simulink model "xtao"  (Simulink 7.0)
settings: Solver=FixedStepDiscrete  SolverMode=SingleTasking  StartTime=0.0  StopTime=inf  FixedStep=0.002  RelTol=1e-3
undefined symbols (not defined in the file): fdesignblkfcn, gcbh, HIL
libraries: dspsigops x27, quarc_library x6
settings Model: Creator=Administrator  LastModifiedBy=Administrator  SimulationMode=external  ExtModeTrigDuration=5000
settings SolverCC: PositivePriorityOrder=on
settings DataIOCC: ExternalInput=[a1, a2]
settings RTWCC: SystemTargetFile=quarc_windows.tlc  TemplateMakefile=quarc_default_tmf  Description=QUARC Win32 Target  ProcessScript=quarc_windows_make_rtw_hook
settings STFCustomTargetCC: TargetPreCompLibLocation=C:\DOCUME~1\ALLUSE~1\APPLIC~1\QUARC\lib\2007b\windows\release  GenFloatMathFcnCalls=ANSI_C  SystemTargetFile=quarc_windows.tlc
settings GRTTargetCC: TargetPreCompLibLocation=C:\DOCUME~1\ALLUSE~1\APPLIC~1\QUARC\lib\2007b\windows\release  CompOptLevelCompliant=off  MatFileLogging=off  ExtMode=on  ExtModeMexFile=quarc_comm

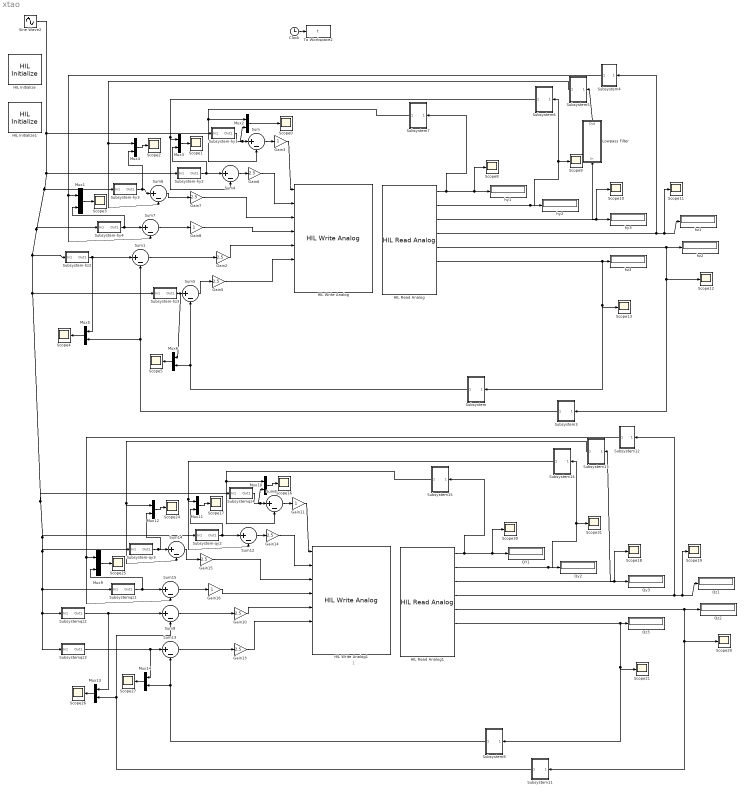
== system xtao ==
  note: 1
  Clock : Clock
      settings: Decimation=10
  Gain{2,5..7,10,13..15} (8 alike) : Gain  Gain=2.5  ParameterDataType=sfix(16)  ParameterScaling=2^0  OutDataType=sfix(16)  OutScaling=2^0
  Gain{3,8,11,16} (4 alike) : Gain  ParameterDataType=sfix(16)  ParameterScaling=2^0  OutDataType=sfix(16)  OutScaling=2^0
  HIL Initialize : quarc_library/Data Acquisition/Generic/Configuration/HIL Initialize  object_name=HIL-1  board_type=qpid  board_number=0  board_options=enc0_dir=0;enc0_filter=1;enc0_a=1;enc0_b=1;enc0_z=0;enc0_reload=0;enc1_dir=0;enc1_filter=1;enc1_a=1;enc1_b=1;enc1_z=0;enc1_reload=0;enc2_dir=0;enc2_filter=1;enc2_a=1;enc2_b=1;enc2_z=0;enc2_reload=0;enc3_dir=0;enc3_filter=1;enc3_a=1;enc3_b=1;enc3_z=0;enc3_reload=0;enc4_dir=0;enc4_filter=1;enc4_a=1;enc4_b=1;enc4_z=0;enc4_reload=0;enc5_dir=0;enc5_filter=1;enc5_a=1;enc5_b=1;enc5_z=0;enc5_reload=0;enc6_dir=0;enc6_filter=1;enc6_a=1;enc6_b=1;enc6_z=0;enc6_reload=0;enc7_dir=0;enc7_filter=1;enc7_a=1;enc7_b=1;enc7_z=0;enc7_reload=0;ext_int_polarity=0;fuse_polarity=0;convert_polarity=0;watchdog_polarity=0;ext_int_watchdog=0;fuse_watchdog=0;trig1_watchdog=0;watchdog_to_trig1=0;watchdog_to_trig2=0;counter_to_trig0=0;trigger_adcs=0;latch_on_adc=0;pwm_immediate=0  exclusive=off  active=off  hardware_clocks=[0:16]  clock_modes=[]  set_clock_params_at_start=off  set_clock_params_at_switch_in=off  analog_input_channels=[0:7]  analog_input_maximums=10  analog_input_minimums=-10  set_analog_input_params_at_start=off  set_analog_input_params_at_switch_in=off  analog_output_channels=[0:7]  analog_output_maximums=10  analog_output_minimums=-10  initial_analog_outputs=[0]  final_analog_outputs=[0]  watchdog_analog_outputs=0  set_analog_output_params_at_start=off  set_analog_output_params_at_switch_in=off  set_analog_outputs_at_start=on  set_analog_outputs_at_switch_in=off  set_analog_outputs_at_terminate=on  set_analog_outputs_at_switch_out=off  set_analog_outputs_on_watchdog=off  digital_input_channels=[]  digital_output_channels=[]  digital_output_configuration=[]  initial_digital_outputs=[1]  final_digital_outputs=[1]  watchdog_digital_outputs=[2]  set_digital_output_params_at_start=off  set_digital_output_params_at_switch_in=off  set_digital_outputs_at_start=on  set_digital_outputs_at_switch_in=off  set_digital_outputs_at_terminate=on  set_digital_outputs_at_switch_out=off  set_digital_outputs_on_watchdog=off  encoder_channels=[0:7]  quadrature=[4]  encoder_filter_frequency=40e6/1  initial_encoder_counts=[0]  set_encoder_params_at_start=on  set_encoder_params_at_switch_in=off  set_encoder_counts_at_start=on  set_encoder_counts_at_switch_in=off  pwm_channels=[0:7]  pwm_modes=0  pwm_frequency=40e6/4095  pwm_configuration=[0]  pwm_alignment=[0]  pwm_polarity=[1]  pwm_leading_deadband=[0]  pwm_trailing_deadband=[0]  initial_pwm_outputs=[0]  final_pwm_outputs=[0]  watchdog_pwm_outputs=[0]  set_pwm_params_at_start=on  set_pwm_params_at_switch_in=off  set_pwm_outputs_at_start=on  set_pwm_outputs_at_switch_in=off  set_pwm_outputs_at_terminate=on  set_pwm_outputs_at_switch_out=off  set_pwm_outputs_on_watchdog=off  other_output_channels=[]  initial_other_outputs=[]  final_other_outputs=[]  watchdog_other_outputs=[]  set_other_outputs_at_start=off  set_other_outputs_at_switch_in=off  set_other_outputs_at_terminate=off  set_other_outputs_at_switch_out=off  set_other_outputs_on_watchdog=off
  HIL Initialize1 : quarc_library/Data Acquisition/Generic/Configuration/HIL Initialize  object_name=HIL-2  board_type=qpid  board_number=1  board_options=enc0_dir=0;enc0_filter=1;enc0_a=1;enc0_b=1;enc0_z=0;enc0_reload=0;enc1_dir=0;enc1_filter=1;enc1_a=1;enc1_b=1;enc1_z=0;enc1_reload=0;enc2_dir=0;enc2_filter=1;enc2_a=1;enc2_b=1;enc2_z=0;enc2_reload=0;enc3_dir=0;enc3_filter=1;enc3_a=1;enc3_b=1;enc3_z=0;enc3_reload=0;enc4_dir=0;enc4_filter=1;enc4_a=1;enc4_b=1;enc4_z=0;enc4_reload=0;enc5_dir=0;enc5_filter=1;enc5_a=1;enc5_b=1;enc5_z=0;enc5_reload=0;enc6_dir=0;enc6_filter=1;enc6_a=1;enc6_b=1;enc6_z=0;enc6_reload=0;enc7_dir=0;enc7_filter=1;enc7_a=1;enc7_b=1;enc7_z=0;enc7_reload=0;ext_int_polarity=0;fuse_polarity=0;convert_polarity=0;watchdog_polarity=0;ext_int_watchdog=0;fuse_watchdog=0;trig1_watchdog=0;watchdog_to_trig1=0;watchdog_to_trig2=0;counter_to_trig0=0;trigger_adcs=0;latch_on_adc=0;pwm_immediate=0  exclusive=off  active=off  hardware_clocks=[0:16]  clock_modes=[]  set_clock_params_at_start=off  set_clock_params_at_switch_in=off  analog_input_channels=[0:7]  analog_input_maximums=10  analog_input_minimums=-10  set_analog_input_params_at_start=off  set_analog_input_params_at_switch_in=off  analog_output_channels=[0:7]  analog_output_maximums=10  analog_output_minimums=-10  initial_analog_outputs=[0]  final_analog_outputs=[0]  watchdog_analog_outputs=0  set_analog_output_params_at_start=off  set_analog_output_params_at_switch_in=off  set_analog_outputs_at_start=on  set_analog_outputs_at_switch_in=off  set_analog_outputs_at_terminate=on  set_analog_outputs_at_switch_out=off  set_analog_outputs_on_watchdog=off  digital_input_channels=[]  digital_output_channels=[]  digital_output_configuration=[]  initial_digital_outputs=[1]  final_digital_outputs=[1]  watchdog_digital_outputs=[2]  set_digital_output_params_at_start=off  set_digital_output_params_at_switch_in=off  set_digital_outputs_at_start=on  set_digital_outputs_at_switch_in=off  set_digital_outputs_at_terminate=on  set_digital_outputs_at_switch_out=off  set_digital_outputs_on_watchdog=off  encoder_channels=[0:7]  quadrature=[4]  encoder_filter_frequency=40e6/1  initial_encoder_counts=[0]  set_encoder_params_at_start=on  set_encoder_params_at_switch_in=off  set_encoder_counts_at_start=on  set_encoder_counts_at_switch_in=off  pwm_channels=[0:7]  pwm_modes=0  pwm_frequency=40e6/4095  pwm_configuration=[0]  pwm_alignment=[0]  pwm_polarity=[1]  pwm_leading_deadband=[0]  pwm_trailing_deadband=[0]  initial_pwm_outputs=[0]  final_pwm_outputs=[0]  watchdog_pwm_outputs=[0]  set_pwm_params_at_start=on  set_pwm_params_at_switch_in=off  set_pwm_outputs_at_start=on  set_pwm_outputs_at_switch_in=off  set_pwm_outputs_at_terminate=on  set_pwm_outputs_at_switch_out=off  set_pwm_outputs_on_watchdog=off  other_output_channels=[]  initial_other_outputs=[]  final_other_outputs=[]  watchdog_other_outputs=[]  set_other_outputs_at_start=off  set_other_outputs_at_switch_in=off  set_other_outputs_at_terminate=off  set_other_outputs_at_switch_out=off  set_other_outputs_on_watchdog=off
  HIL Read Analog : quarc_library/Data Acquisition/Generic/Immediate I//O/HIL Read Analog  object_name=HIL-2  channels=[0:7]  sample_time=qc_get_step_size  active=on  vector_output=off
  HIL Read Analog1 : quarc_library/Data Acquisition/Generic/Immediate I//O/HIL Read Analog  object_name=HIL-1  channels=[0:7]  sample_time=qc_get_step_size  active=on  vector_output=off
  HIL Write Analog : quarc_library/Data Acquisition/Generic/Immediate I//O/HIL Write Analog  object_name=HIL-2  channels=[0:7]  sample_time=-1  active=off  vector_input=off
  HIL Write Analog1 : quarc_library/Data Acquisition/Generic/Immediate I//O/HIL Write Analog  object_name=HIL-1  channels=[0:7]  sample_time=-1  active=off  vector_input=off
  Lowpass Filter : Subsystem  Orientation=up  DialogController=fdesignblkfcn  DialogControllerArgs=DataTag7  InitFcn=fdesignblkfcn(gcbh, {'InitFcn'});
      settings: CopyFcn=fdesignblkfcn(gcbh, {'CopyFcn'});
      mask Type: Lowpass Filter
      mask Description: Design a lowpass filter
      mask Help: helpview(mapfilelocation('dspblks'), 'dsplowpassfilter')
      mask Display: disp('Lowpass')
  Mux{1..4,9..12} (8 alike) : Mux  Inputs=2
  Mux{5..6,13..14} (4 alike) : Mux  Orientation=left  Inputs=2
  QY1 : Display
  Qy2 : Display
  Qy3 : Display
  Qz1 : Display
  Qz2 : Display
  Qz3 : Display
  Scope{0..5,8..13,16..21,24..27,30..31} (24 alike) : Scope
      Scope0 settings: TimeRange=15  YMin=2  YMax=5.75  SaveName=ScopeData3  SampleInput=on
      Scope1 settings: TimeRange=15  YMin=0.5  YMax=4  SaveName=ScopeData4  SampleInput=on
      Scope10 settings: YMin=0.6  YMax=1.45  SaveName=ScopeData11
      Scope11 settings: YMin=1.045  YMax=1.065  SaveName=ScopeData2
      Scope12 settings: YMin=0.68175  YMax=0.68375  SaveName=ScopeData12
      Scope13 settings: YMin=0  YMax=2  SaveName=ScopeData13
      Scope16 settings: TimeRange=15  YMin=0.5  YMax=4.5  SaveName=ScopeData16  SampleInput=on
      Scope17 settings: TimeRange=15  YMin=0.5  YMax=4  SaveName=ScopeData17  SampleInput=on
      Scope18 settings: YMin=0.5  YMax=0.85  SaveName=ScopeData18
      Scope19 settings: YMin=0.7  YMax=1.3  SaveName=ScopeData19
      Scope2 settings: TimeRange=15  YMin=-0.5  YMax=5.25  SaveName=ScopeData5  SampleInput=on
      Scope20 settings: YMin=0.4  YMax=1.3  SaveName=ScopeData20
      Scope21 settings: YMin=0  YMax=2  SaveName=ScopeData21
      Scope24 settings: TimeRange=15  YMin=0.2  YMax=2.4  SaveName=ScopeData24  SampleInput=on
      Scope25 settings: TimeRange=15  YMin=0.3  YMax=2.1  SaveName=ScopeData25  SampleInput=on
      Scope26 settings: TimeRange=15  YMax=10  SaveName=ScopeData26  SampleInput=on
      Scope27 settings: TimeRange=15  YMin=1.975  YMax=2.4  SaveName=ScopeData27  SampleInput=on
      Scope3 settings: TimeRange=15  YMin=1.85  YMax=2.3  SampleInput=on
      Scope30 settings: YMin=-0.005  YMax=0.015  SaveName=ScopeData30
      Scope31 settings: YMin=-0.000305176  YMax=-0.000305176  SaveName=ScopeData31
      Scope4 settings: TimeRange=15  YMin=0.5  YMax=4  SaveName=ScopeData6  SampleInput=on
      Scope5 settings: TimeRange=15  YMin=-2.75  YMax=3  SaveName=ScopeData7  SampleInput=on
      Scope8 settings: TimeRange=10  YMin=0.8785  YMax=0.8875  SaveName=ScopeData9
      Scope9 settings: YMin=0.129  YMax=0.1307  SaveName=ScopeData10
  Sine Wave2 : Sin  Bias=20  Frequency=3.14  SampleTime=0
  Subsystem : Subsystem  Orientation=left
  Subsystem-hy1 : Subsystem
  Subsystem-hy2 : Subsystem
  Subsystem-hy3 : Subsystem
  Subsystem-hy4 : Subsystem
  Subsystem-hz2 : Subsystem
  Subsystem-hz3 : Subsystem
  Subsystem-qy2 : Subsystem
  Subsystem-qy3 : Subsystem
  Subsystem11 : Subsystem  Orientation=left
  Subsystem12 : Subsystem  Orientation=left
  Subsystem13 : Subsystem  Orientation=left
  Subsystem14 : Subsystem  Orientation=left
  Subsystem15 : Subsystem  Orientation=left
  Subsystem3 : Subsystem  Orientation=left
  Subsystem4 : Subsystem  Orientation=left
  Subsystem5 : Subsystem  Orientation=left
  Subsystem6 : Subsystem  Orientation=left
  Subsystem7 : Subsystem  Orientation=left
  Subsystem8 : Subsystem  Orientation=left
  Subsystemqz1 : Subsystem
  Subsystemqz2 : Subsystem
  Subsystemqz3 : Subsystem
  Subsystemqz4 : Subsystem
  Sum{,1,4..9,12..15} (12 alike) : Sum  Inputs=|+-  OutDataType=sfix(16)  OutScaling=2^0
  To Workspace2 : ToWorkspace  VariableName=t  SampleTime=-1  SaveFormat=Array
  hy1 : Display
  hy2 : Display
  hy3 : Display
  hz1 : Display
  hz2 : Display
  hz3 : Display
  wires:
  HIL Read Analog/1 -> Subsystem7/1(In1), hy1/1, Scope8/1
  HIL Read Analog/2 -> hy2/1, Subsystem6/1(In1), Scope9/1
  HIL Read Analog/3 -> hy3/1, Scope10/1, Lowpass Filter/1(In)
  HIL Read Analog/4 -> Subsystem4/1(In1), hz1/1, Scope11/1
  HIL Read Analog/5 -> hz2/1, Scope12/1, Subsystem3/1(In1)
  HIL Read Analog/6 -> hz3/1, Subsystem/1(In1), Scope13/1
  Gain8/1 -> HIL Write Analog/4
  Clock/1 -> To Workspace2/1
  Gain2/1 -> HIL Write Analog/5
  Gain5/1 -> HIL Write Analog/6
  Sum5/1 -> Gain5/1
  Subsystem/1(Out1) -> Sum5/2, Mux6/2
  Sum1/1 -> Gain2/1
  Subsystem3/1(Out1) -> Sum1/2, Mux5/2
  Sum/1 -> Gain3/1
  Subsystem-hy1/1(Out1) -> Sum/1, Mux2/2
  Sum4/1 -> Gain6/1
  Subsystem-hy2/1(Out1) -> Sum4/1, Mux3/2
  Sum6/1 -> Gain7/1
  Subsystem7/1(Out1) -> Sum/2, Mux2/1
  Subsystem6/1(Out1) -> Sum4/2, Mux3/1
  Subsystem5/1(Out1) -> Sum6/2, Mux4/1
  Subsystem4/1(Out1) -> Sum7/2, Mux1/1
  Sum7/1 -> Gain8/1
  Subsystem-hy4/1(Out1) -> Sum7/1, Mux1/2
  Mux1/1 -> Scope3/1
  Subsystem-hz2/1(Out1) -> Sum1/1, Mux5/1
  Subsystem-hz3/1(Out1) -> Sum5/1, Mux6/1
  Mux2/1 -> Scope0/1
  Gain3/1 -> HIL Write Analog/1
  Mux3/1 -> Scope1/1
  Mux4/1 -> Scope2/1
  Mux5/1 -> Scope4/1
  Mux6/1 -> Scope5/1
  HIL Read Analog1/1 -> Subsystem15/1(In1), QY1/1, Scope30/1
  HIL Read Analog1/2 -> Qy2/1, Subsystem14/1(In1), Scope31/1
  HIL Read Analog1/3 -> Qy3/1, Subsystem13/1(In1), Scope18/1
  HIL Read Analog1/4 -> Subsystem12/1(In1), Qz1/1, Scope19/1
  HIL Read Analog1/5 -> Qz2/1, Scope20/1, Subsystem11/1(In1)
  HIL Read Analog1/6 -> Qz3/1, Subsystem8/1(In1), Scope21/1
  Gain16/1 -> HIL Write Analog1/4
  Gain10/1 -> HIL Write Analog1/5
  Gain14/1 -> HIL Write Analog1/2
  Gain13/1 -> HIL Write Analog1/6
  Sum13/1 -> Gain13/1
  Subsystem8/1(Out1) -> Sum13/2, Mux14/2
  Sum9/1 -> Gain10/1
  Subsystem11/1(Out1) -> Sum9/2, Mux13/2
  Sum8/1 -> Gain11/1
  Subsystemqz4/1(Out1) -> Sum8/1, Mux10/2
  Sum12/1 -> Gain14/1
  Subsystem-qy2/1(Out1) -> Sum12/1, Mux11/2
  Sum14/1 -> Gain15/1
  Subsystem-qy3/1(Out1) -> Mux12/2, Sum14/1
  Subsystem15/1(Out1) -> Sum8/2, Mux10/1
  Subsystem14/1(Out1) -> Sum12/2, Mux11/1
  Subsystem13/1(Out1) -> Sum14/2, Mux12/1
  Subsystem12/1(Out1) -> Sum15/2, Mux9/1
  Sum15/1 -> Gain16/1
  Subsystemqz1/1(Out1) -> Sum15/1, Mux9/2
  Mux9/1 -> Scope25/1
  Subsystemqz2/1(Out1) -> Sum9/1, Mux13/1
  Subsystemqz3/1(Out1) -> Mux14/1, Sum13/1
  Mux10/1 -> Scope16/1
  Gain11/1 -> HIL Write Analog1/1
  Mux11/1 -> Scope17/1
  Mux12/1 -> Scope24/1
  Mux13/1 -> Scope26/1
  Mux14/1 -> Scope27/1
  Lowpass Filter/1(Out) -> Subsystem5/1(In1)
  Sine Wave2/1 -> Subsystem-hy2/1(In1), Subsystem-hy3/1(In1), Subsystem-hz2/1(In1), Subsystem-hz3/1(In1), Subsystem-qy2/1(In1), Subsystem-qy3/1(In1), Subsystemqz2/1(In1), Subsystemqz3/1(In1), Subsystemqz1/1(In1), Subsystemqz4/1(In1), Subsystem-hy4/1(In1), Subsystem-hy1/1(In1)
  Subsystem-hy3/1(Out1) -> Sum6/1, Mux4/2
  Gain15/1 -> HIL Write Analog1/3
  Gain6/1 -> HIL Write Analog/2
  Gain7/1 -> HIL Write Analog/3

== system xtao/Lowpass Filter ==
  In : Inport  OutDataType=sfix(16)  OutScaling=2^0
  Generated Filter Block : Subsystem  Tag=FilterWizardSubSystem
      settings: ErrorFcn=dspFilterRealizedInBasicElemsAlgLoopErrFcnCallback
  Out : Outport  OutDataType=sfix(16)  OutScaling=2^0
  wires:
  In/1 -> Generated Filter Block/1(Input)
  Generated Filter Block/1(Output) -> Out/1

== system xtao/Subsystem ==
  In1 : Inport  Orientation=left
  Constant9 : Constant  Orientation=left  Value=-3.9461  OutDataType=sfix(16)  OutScaling=2^0
  Gain4 : Gain  Orientation=left  Gain=6.2956  ParameterDataType=sfix(16)  ParameterScaling=2^0  OutDataType=sfix(16)  OutScaling=2^0
  Sum4 : Sum  Orientation=left  Inputs=|++  OutDataType=sfix(16)  OutScaling=2^0
  Out1 : Outport  Orientation=left
  wires:
  Constant9/1 -> Sum4/1
  Gain4/1 -> Sum4/2
  In1/1 -> Gain4/1
  Sum4/1 -> Out1/1

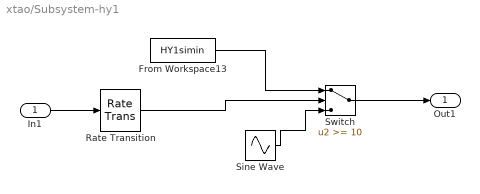
== system xtao/Subsystem-hy1 ==
  In1 : Inport  OutDataType=sfix(16)  OutScaling=2^0
  From Workspace13 : FromWorkspace  VariableName=HY1simin  SampleTime=0.01  Interpolate=off  OutputAfterFinalValue=Cyclic repetition
  Rate Transition : RateTransition
  Sine Wave : Sin  Amplitude=2.5  Bias=2.5  Frequency=3.14  SampleTime=0
  Switch : Switch  Threshold=10  OutDataType=sfix(16)  OutScaling=2^0
  Out1 : Outport  OutDataType=sfix(16)  OutScaling=2^0
  wires:
  From Workspace13/1 -> Switch/1
  Rate Transition/1 -> Switch/2
  Switch/1 -> Out1/1
  In1/1 -> Rate Transition/1
  Sine Wave/1 -> Switch/3

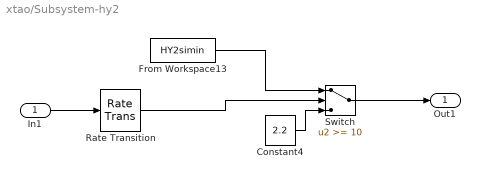
== system xtao/Subsystem-hy2 ==
  In1 : Inport  OutDataType=sfix(16)  OutScaling=2^0
  Constant4 : Constant  Value=2.2  OutDataType=sfix(16)  OutScaling=2^0
  From Workspace13 : FromWorkspace  VariableName=HY2simin  SampleTime=0.01  Interpolate=off  OutputAfterFinalValue=Cyclic repetition
  Rate Transition : RateTransition
  Switch : Switch  Threshold=10  OutDataType=sfix(16)  OutScaling=2^0
  Out1 : Outport  OutDataType=sfix(16)  OutScaling=2^0
  wires:
  From Workspace13/1 -> Switch/1
  Rate Transition/1 -> Switch/2
  Switch/1 -> Out1/1
  In1/1 -> Rate Transition/1
  Constant4/1 -> Switch/3

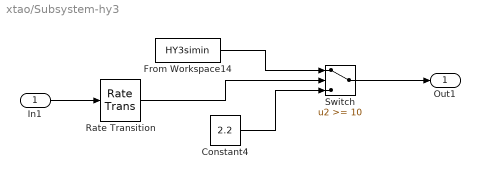
== system xtao/Subsystem-hy3 ==
  In1 : Inport  OutDataType=sfix(16)  OutScaling=2^0
  Constant4 : Constant  Value=2.2  OutDataType=sfix(16)  OutScaling=2^0
  From Workspace14 : FromWorkspace  VariableName=HY3simin  SampleTime=0.01  Interpolate=off  OutputAfterFinalValue=Cyclic repetition
  Rate Transition : RateTransition
  Switch : Switch  Threshold=10  OutDataType=sfix(16)  OutScaling=2^0
  Out1 : Outport  OutDataType=sfix(16)  OutScaling=2^0
  wires:
  Constant4/1 -> Switch/3
  From Workspace14/1 -> Switch/1
  Rate Transition/1 -> Switch/2
  Switch/1 -> Out1/1
  In1/1 -> Rate Transition/1

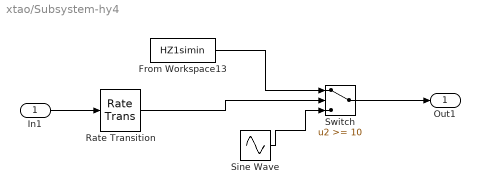
== system xtao/Subsystem-hy4 ==
  In1 : Inport  OutDataType=sfix(16)  OutScaling=2^0
  From Workspace13 : FromWorkspace  VariableName=HZ1simin  SampleTime=0.01  Interpolate=off  OutputAfterFinalValue=Cyclic repetition
  Rate Transition : RateTransition
  Sine Wave : Sin  Amplitude=2.5  Bias=2.5  Frequency=3.14  SampleTime=0
  Switch : Switch  Threshold=10  OutDataType=sfix(16)  OutScaling=2^0
  Out1 : Outport  OutDataType=sfix(16)  OutScaling=2^0
  wires:
  From Workspace13/1 -> Switch/1
  Rate Transition/1 -> Switch/2
  Switch/1 -> Out1/1
  In1/1 -> Rate Transition/1
  Sine Wave/1 -> Switch/3

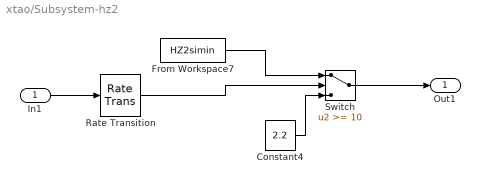
== system xtao/Subsystem-hz2 ==
  In1 : Inport  OutDataType=sfix(16)  OutScaling=2^0
  Constant4 : Constant  Value=2.2  OutDataType=sfix(16)  OutScaling=2^0
  From Workspace7 : FromWorkspace  VariableName=HZ2simin  SampleTime=0.01  Interpolate=off  OutputAfterFinalValue=Cyclic repetition
  Rate Transition : RateTransition
  Switch : Switch  Threshold=10  OutDataType=sfix(16)  OutScaling=2^0
  Out1 : Outport  OutDataType=sfix(16)  OutScaling=2^0
  wires:
  From Workspace7/1 -> Switch/1
  Rate Transition/1 -> Switch/2
  Switch/1 -> Out1/1
  In1/1 -> Rate Transition/1
  Constant4/1 -> Switch/3

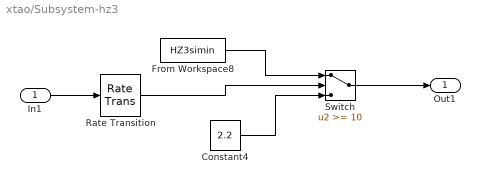
== system xtao/Subsystem-hz3 ==
  In1 : Inport  OutDataType=sfix(16)  OutScaling=2^0
  Constant4 : Constant  Value=2.2  OutDataType=sfix(16)  OutScaling=2^0
  From Workspace8 : FromWorkspace  VariableName=HZ3simin  SampleTime=0.01  Interpolate=off  OutputAfterFinalValue=Cyclic repetition
  Rate Transition : RateTransition
  Switch : Switch  Threshold=10  OutDataType=sfix(16)  OutScaling=2^0
  Out1 : Outport  OutDataType=sfix(16)  OutScaling=2^0
  wires:
  Constant4/1 -> Switch/3
  From Workspace8/1 -> Switch/1
  Rate Transition/1 -> Switch/2
  Switch/1 -> Out1/1
  In1/1 -> Rate Transition/1

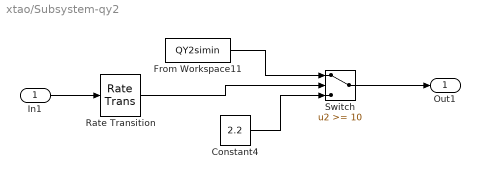
== system xtao/Subsystem-qy2 ==
  In1 : Inport  OutDataType=sfix(16)  OutScaling=2^0
  Constant4 : Constant  Value=2.2  OutDataType=sfix(16)  OutScaling=2^0
  From Workspace11 : FromWorkspace  VariableName=QY2simin  SampleTime=0.01  Interpolate=off  OutputAfterFinalValue=Cyclic repetition
  Rate Transition : RateTransition
  Switch : Switch  Threshold=10  OutDataType=sfix(16)  OutScaling=2^0
  Out1 : Outport  OutDataType=sfix(16)  OutScaling=2^0
  wires:
  Rate Transition/1 -> Switch/2
  Switch/1 -> Out1/1
  In1/1 -> Rate Transition/1
  From Workspace11/1 -> Switch/1
  Constant4/1 -> Switch/3

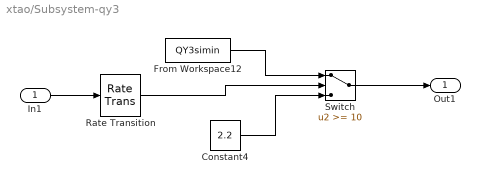
== system xtao/Subsystem-qy3 ==
  In1 : Inport  OutDataType=sfix(16)  OutScaling=2^0
  Constant4 : Constant  Value=2.2  OutDataType=sfix(16)  OutScaling=2^0
  From Workspace12 : FromWorkspace  VariableName=QY3simin  SampleTime=0.01  Interpolate=off  OutputAfterFinalValue=Cyclic repetition
  Rate Transition : RateTransition
  Switch : Switch  Threshold=10  OutDataType=sfix(16)  OutScaling=2^0
  Out1 : Outport  OutDataType=sfix(16)  OutScaling=2^0
  wires:
  Constant4/1 -> Switch/3
  From Workspace12/1 -> Switch/1
  Rate Transition/1 -> Switch/2
  Switch/1 -> Out1/1
  In1/1 -> Rate Transition/1

== system xtao/Subsystem11 ==
  In1 : Inport  Orientation=left
  Constant9 : Constant  Orientation=left  Value=-4.0345  OutDataType=sfix(16)  OutScaling=2^0
  Gain4 : Gain  Orientation=left  Gain=7.5666  ParameterDataType=sfix(16)  ParameterScaling=2^0  OutDataType=sfix(16)  OutScaling=2^0
  Sum4 : Sum  Orientation=left  Inputs=|++  OutDataType=sfix(16)  OutScaling=2^0
  Out1 : Outport  Orientation=left
  wires:
  Constant9/1 -> Sum4/1
  Gain4/1 -> Sum4/2
  In1/1 -> Gain4/1
  Sum4/1 -> Out1/1

== system xtao/Subsystem12 ==
  In1 : Inport  Orientation=left
  Constant9 : Constant  Orientation=left  Value=44.9691  OutDataType=sfix(16)  OutScaling=2^0
  Gain4 : Gain  Orientation=left  Gain=-10.3093  ParameterDataType=sfix(16)  ParameterScaling=2^0  OutDataType=sfix(16)  OutScaling=2^0
  Sum4 : Sum  Orientation=left  Inputs=|++  OutDataType=sfix(16)  OutScaling=2^0
  Out1 : Outport  Orientation=left
  wires:
  Constant9/1 -> Sum4/1
  Gain4/1 -> Sum4/2
  In1/1 -> Gain4/1
  Sum4/1 -> Out1/1

== system xtao/Subsystem13 ==
  In1 : Inport  Orientation=left
  Constant9 : Constant  Orientation=left  Value=-3.3411  OutDataType=sfix(16)  OutScaling=2^0
  Gain4 : Gain  Orientation=left  Gain=6.6836  ParameterDataType=sfix(16)  ParameterScaling=2^0  OutDataType=sfix(16)  OutScaling=2^0
  Sum4 : Sum  Orientation=left  Inputs=|++  OutDataType=sfix(16)  OutScaling=2^0
  Out1 : Outport  Orientation=left
  wires:
  Constant9/1 -> Sum4/1
  Gain4/1 -> Sum4/2
  In1/1 -> Gain4/1
  Sum4/1 -> Out1/1

== system xtao/Subsystem14 ==
  In1 : Inport  Orientation=left
  Constant9 : Constant  Orientation=left  Value=-3.8142  OutDataType=sfix(16)  OutScaling=2^0
  Gain4 : Gain  Orientation=left  Gain=7.9479  ParameterDataType=sfix(16)  ParameterScaling=2^0  OutDataType=sfix(16)  OutScaling=2^0
  Sum4 : Sum  Orientation=left  Inputs=|++  OutDataType=sfix(16)  OutScaling=2^0
  Out1 : Outport  Orientation=left
  wires:
  Constant9/1 -> Sum4/1
  Gain4/1 -> Sum4/2
  In1/1 -> Gain4/1
  Sum4/1 -> Out1/1

== system xtao/Subsystem15 ==
  In1 : Inport  Orientation=left
  Constant9 : Constant  Orientation=left  Value=-3.4379  OutDataType=sfix(16)  OutScaling=2^0
  Gain4 : Gain  Orientation=left  Gain=8.6655  ParameterDataType=sfix(16)  ParameterScaling=2^0  OutDataType=sfix(16)  OutScaling=2^0
  Sum4 : Sum  Orientation=left  Inputs=|++  OutDataType=sfix(16)  OutScaling=2^0
  Out1 : Outport  Orientation=left
  wires:
  Constant9/1 -> Sum4/1
  Gain4/1 -> Sum4/2
  In1/1 -> Gain4/1
  Sum4/1 -> Out1/1

== system xtao/Subsystem3 ==
  In1 : Inport  Orientation=left
  Constant9 : Constant  Orientation=left  Value=-3.8231  OutDataType=sfix(16)  OutScaling=2^0
  Gain4 : Gain  Orientation=left  Gain=6.6489  ParameterDataType=sfix(16)  ParameterScaling=2^0  OutDataType=sfix(16)  OutScaling=2^0
  Sum4 : Sum  Orientation=left  Inputs=|++  OutDataType=sfix(16)  OutScaling=2^0
  Out1 : Outport  Orientation=left
  wires:
  Constant9/1 -> Sum4/1
  Gain4/1 -> Sum4/2
  In1/1 -> Gain4/1
  Sum4/1 -> Out1/1

== system xtao/Subsystem4 ==
  In1 : Inport  Orientation=left
  Constant9 : Constant  Orientation=left  Value=46.9136  OutDataType=sfix(16)  OutScaling=2^0
  Gain4 : Gain  Orientation=left  Gain=-10.2881  ParameterDataType=sfix(16)  ParameterScaling=2^0  OutDataType=sfix(16)  OutScaling=2^0
  Sum4 : Sum  Orientation=left  Inputs=|++  OutDataType=sfix(16)  OutScaling=2^0
  Out1 : Outport  Orientation=left
  wires:
  Constant9/1 -> Sum4/1
  Gain4/1 -> Sum4/2
  In1/1 -> Gain4/1
  Sum4/1 -> Out1/1

== system xtao/Subsystem5 ==
  In1 : Inport  Orientation=left
  Constant9 : Constant  Orientation=left  Value=-3.7624  OutDataType=sfix(16)  OutScaling=2^0
  Gain4 : Gain  Orientation=left  Gain=6.2189  ParameterDataType=sfix(16)  ParameterScaling=2^0  OutDataType=sfix(16)  OutScaling=2^0
  Sum4 : Sum  Orientation=left  Inputs=|++  OutDataType=sfix(16)  OutScaling=2^0
  Out1 : Outport  Orientation=left
  wires:
  Constant9/1 -> Sum4/1
  Gain4/1 -> Sum4/2
  In1/1 -> Gain4/1
  Sum4/1 -> Out1/1

== system xtao/Subsystem6 ==
  In1 : Inport  Orientation=left
  Constant9 : Constant  Orientation=left  Value=-4.6642  OutDataType=sfix(16)  OutScaling=2^0
  Gain4 : Gain  Orientation=left  Gain=7.4627  ParameterDataType=sfix(16)  ParameterScaling=2^0  OutDataType=sfix(16)  OutScaling=2^0
  Sum4 : Sum  Orientation=left  Inputs=|++  OutDataType=sfix(16)  OutScaling=2^0
  Out1 : Outport  Orientation=left
  wires:
  Constant9/1 -> Sum4/1
  Gain4/1 -> Sum4/2
  In1/1 -> Gain4/1
  Sum4/1 -> Out1/1

== system xtao/Subsystem7 ==
  In1 : Inport  Orientation=left
  Constant9 : Constant  Orientation=left  Value=-5.1224  OutDataType=sfix(16)  OutScaling=2^0
  Gain4 : Gain  Orientation=left  Gain=8.7413  ParameterDataType=sfix(16)  ParameterScaling=2^0  OutDataType=sfix(16)  OutScaling=2^0
  Sum4 : Sum  Orientation=left  Inputs=|++  OutDataType=sfix(16)  OutScaling=2^0
  Out1 : Outport  Orientation=left
  wires:
  Constant9/1 -> Sum4/1
  Gain4/1 -> Sum4/2
  In1/1 -> Gain4/1
  Sum4/1 -> Out1/1

== system xtao/Subsystem8 ==
  In1 : Inport  Orientation=left
  Constant9 : Constant  Orientation=left  Value=-3.1294  OutDataType=sfix(16)  OutScaling=2^0
  Gain4 : Gain  Orientation=left  Gain=6.7240  ParameterDataType=sfix(16)  ParameterScaling=2^0  OutDataType=sfix(16)  OutScaling=2^0
  Sum4 : Sum  Orientation=left  Inputs=|++  OutDataType=sfix(16)  OutScaling=2^0
  Out1 : Outport  Orientation=left
  wires:
  Constant9/1 -> Sum4/1
  Gain4/1 -> Sum4/2
  In1/1 -> Gain4/1
  Sum4/1 -> Out1/1

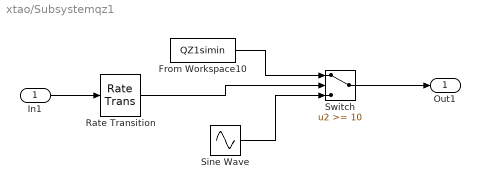
== system xtao/Subsystemqz1 ==
  In1 : Inport  OutDataType=sfix(16)  OutScaling=2^0
  From Workspace10 : FromWorkspace  VariableName=QZ1simin  SampleTime=0.01  Interpolate=off  OutputAfterFinalValue=Cyclic repetition
  Rate Transition : RateTransition
  Sine Wave : Sin  Amplitude=2.5  Bias=2.5  Frequency=3.14  SampleTime=0
  Switch : Switch  Threshold=10  OutDataType=sfix(16)  OutScaling=2^0
  Out1 : Outport  OutDataType=sfix(16)  OutScaling=2^0
  wires:
  Sine Wave/1 -> Switch/3
  From Workspace10/1 -> Switch/1
  Rate Transition/1 -> Switch/2
  Switch/1 -> Out1/1
  In1/1 -> Rate Transition/1

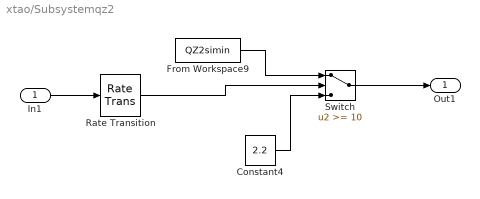
== system xtao/Subsystemqz2 ==
  In1 : Inport  OutDataType=sfix(16)  OutScaling=2^0
  Constant4 : Constant  Value=2.2  OutDataType=sfix(16)  OutScaling=2^0
  From Workspace9 : FromWorkspace  VariableName=QZ2simin  SampleTime=0.01  Interpolate=off  OutputAfterFinalValue=Cyclic repetition
  Rate Transition : RateTransition
  Switch : Switch  Threshold=10  OutDataType=sfix(16)  OutScaling=2^0
  Out1 : Outport  OutDataType=sfix(16)  OutScaling=2^0
  wires:
  From Workspace9/1 -> Switch/1
  Rate Transition/1 -> Switch/2
  Switch/1 -> Out1/1
  In1/1 -> Rate Transition/1
  Constant4/1 -> Switch/3

== system xtao/Subsystemqz3 ==
  In1 : Inport  OutDataType=sfix(16)  OutScaling=2^0
  Constant4 : Constant  Value=2.2  OutDataType=sfix(16)  OutScaling=2^0
  From Workspace10 : FromWorkspace  VariableName=QZ3simin  SampleTime=0.01  Interpolate=off  OutputAfterFinalValue=Cyclic repetition
  Rate Transition : RateTransition
  Switch : Switch  Threshold=10  OutDataType=sfix(16)  OutScaling=2^0
  Out1 : Outport  OutDataType=sfix(16)  OutScaling=2^0
  wires:
  Constant4/1 -> Switch/3
  From Workspace10/1 -> Switch/1
  Rate Transition/1 -> Switch/2
  Switch/1 -> Out1/1
  In1/1 -> Rate Transition/1

== system xtao/Subsystemqz4 ==
  In1 : Inport  OutDataType=sfix(16)  OutScaling=2^0
  From Workspace10 : FromWorkspace  VariableName=QY1simin  SampleTime=0.01  Interpolate=off  OutputAfterFinalValue=Cyclic repetition
  Rate Transition : RateTransition
  Sine Wave : Sin  Amplitude=2.5  Bias=2.5  Frequency=3.14  SampleTime=0
  Switch : Switch  Threshold=10  OutDataType=sfix(16)  OutScaling=2^0
  Out1 : Outport  OutDataType=sfix(16)  OutScaling=2^0
  wires:
  In1/1 -> Rate Transition/1
  Switch/1 -> Out1/1
  Rate Transition/1 -> Switch/2
  From Workspace10/1 -> Switch/1
  Sine Wave/1 -> Switch/3

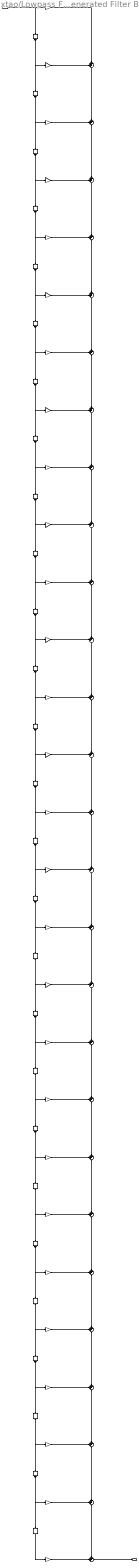
== system xtao/Lowpass Filter/Generated Filter Block ==
  Input : Inport
  BodyDelay{2..28} (27 alike) : dspsigops/Delay  Orientation=down  dly_unit=Samples  delay=1  ic_detail=off  dif_ic_for_ch=off  dif_ic_for_dly=off  ic=0  reset_popup=None
  BodyLSum{2..27} (26 alike) : Sum  Orientation=down  Inputs=++|  OutScaling=1  RndMeth=Nearest  SaturateOnIntegerOverflow=on
  BodyLSum28 : Sum  Inputs=++|  OutScaling=1  RndMeth=Nearest  SaturateOnIntegerOverflow=on
  b(1) : Gain  Gain=0.0030532375936556358  ParameterDataTypeMode=Specify via dialog  ParameterDataType=float('double')  ParameterScalingMode=Use specified scaling  ParameterScaling=1  OutScaling=1  RndMeth=Nearest  SaturateOnIntegerOverflow=on
  b(10) : Gain  Gain=-0.051710781607074402  ParameterDataTypeMode=Specify via dialog  ParameterDataType=float('double')  ParameterScalingMode=Use specified scaling  ParameterScaling=1  OutScaling=1  RndMeth=Nearest  SaturateOnIntegerOverflow=on
  b(11) : Gain  Gain=-0.071497034579946883  ParameterDataTypeMode=Specify via dialog  ParameterDataType=float('double')  ParameterScalingMode=Use specified scaling  ParameterScaling=1  OutScaling=1  RndMeth=Nearest  SaturateOnIntegerOverflow=on
  b(12) : Gain  Gain=0.021409500242294495  ParameterDataTypeMode=Specify via dialog  ParameterDataType=float('double')  ParameterScalingMode=Use specified scaling  ParameterScaling=1  OutScaling=1  RndMeth=Nearest  SaturateOnIntegerOverflow=on
  b(13) : Gain  Gain=0.20428929463408604  ParameterDataTypeMode=Specify via dialog  ParameterDataType=float('double')  ParameterScalingMode=Use specified scaling  ParameterScaling=1  OutScaling=1  RndMeth=Nearest  SaturateOnIntegerOverflow=on
  b(14) : Gain  Gain=0.3545770243381996  ParameterDataTypeMode=Specify via dialog  ParameterDataType=float('double')  ParameterScalingMode=Use specified scaling  ParameterScaling=1  OutScaling=1  RndMeth=Nearest  SaturateOnIntegerOverflow=on
  b(15) : Gain  Gain=0.3545770243381996  ParameterDataTypeMode=Specify via dialog  ParameterDataType=float('double')  ParameterScalingMode=Use specified scaling  ParameterScaling=1  OutScaling=1  RndMeth=Nearest  SaturateOnIntegerOverflow=on
  b(16) : Gain  Gain=0.20428929463408604  ParameterDataTypeMode=Specify via dialog  ParameterDataType=float('double')  ParameterScalingMode=Use specified scaling  ParameterScaling=1  OutScaling=1  RndMeth=Nearest  SaturateOnIntegerOverflow=on
  b(17) : Gain  Gain=0.021409500242294495  ParameterDataTypeMode=Specify via dialog  ParameterDataType=float('double')  ParameterScalingMode=Use specified scaling  ParameterScaling=1  OutScaling=1  RndMeth=Nearest  SaturateOnIntegerOverflow=on
  b(18) : Gain  Gain=-0.071497034579946883  ParameterDataTypeMode=Specify via dialog  ParameterDataType=float('double')  ParameterScalingMode=Use specified scaling  ParameterScaling=1  OutScaling=1  RndMeth=Nearest  SaturateOnIntegerOverflow=on
  b(19) : Gain  Gain=-0.051710781607074402  ParameterDataTypeMode=Specify via dialog  ParameterDataType=float('double')  ParameterScalingMode=Use specified scaling  ParameterScaling=1  OutScaling=1  RndMeth=Nearest  SaturateOnIntegerOverflow=on
  b(2) : Gain  Gain=0.0066380134927875832  ParameterDataTypeMode=Specify via dialog  ParameterDataType=float('double')  ParameterScalingMode=Use specified scaling  ParameterScaling=1  OutScaling=1  RndMeth=Nearest  SaturateOnIntegerOverflow=on
  b(20) : Gain  Gain=0.0090330088298889565  ParameterDataTypeMode=Specify via dialog  ParameterDataType=float('double')  ParameterScalingMode=Use specified scaling  ParameterScaling=1  OutScaling=1  RndMeth=Nearest  SaturateOnIntegerOverflow=on
  b(21) : Gain  Gain=0.034704857949413304  ParameterDataTypeMode=Specify via dialog  ParameterDataType=float('double')  ParameterScalingMode=Use specified scaling  ParameterScaling=1  OutScaling=1  RndMeth=Nearest  SaturateOnIntegerOverflow=on
  b(22) : Gain  Gain=0.013219031256279611  ParameterDataTypeMode=Specify via dialog  ParameterDataType=float('double')  ParameterScalingMode=Use specified scaling  ParameterScaling=1  OutScaling=1  RndMeth=Nearest  SaturateOnIntegerOverflow=on
  b(23) : Gain  Gain=-0.017112476184483319  ParameterDataTypeMode=Specify via dialog  ParameterDataType=float('double')  ParameterScalingMode=Use specified scaling  ParameterScaling=1  OutScaling=1  RndMeth=Nearest  SaturateOnIntegerOverflow=on
  b(24) : Gain  Gain=-0.024022228586093927  ParameterDataTypeMode=Specify via dialog  ParameterDataType=float('double')  ParameterScalingMode=Use specified scaling  ParameterScaling=1  OutScaling=1  RndMeth=Nearest  SaturateOnIntegerOverflow=on
  b(25) : Gain  Gain=-0.010230117696056244  ParameterDataTypeMode=Specify via dialog  ParameterDataType=float('double')  ParameterScalingMode=Use specified scaling  ParameterScaling=1  OutScaling=1  RndMeth=Nearest  SaturateOnIntegerOverflow=on
  b(26) : Gain  Gain=0.0036501248931968783  ParameterDataTypeMode=Specify via dialog  ParameterDataType=float('double')  ParameterScalingMode=Use specified scaling  ParameterScaling=1  OutScaling=1  RndMeth=Nearest  SaturateOnIntegerOverflow=on
  b(27) : Gain  Gain=0.0066380134927875832  ParameterDataTypeMode=Specify via dialog  ParameterDataType=float('double')  ParameterScalingMode=Use specified scaling  ParameterScaling=1  OutScaling=1  RndMeth=Nearest  SaturateOnIntegerOverflow=on
  b(28) : Gain  Gain=0.0030532375936556358  ParameterDataTypeMode=Specify via dialog  ParameterDataType=float('double')  ParameterScalingMode=Use specified scaling  ParameterScaling=1  OutScaling=1  RndMeth=Nearest  SaturateOnIntegerOverflow=on
  b(3) : Gain  Gain=0.0036501248931968783  ParameterDataTypeMode=Specify via dialog  ParameterDataType=float('double')  ParameterScalingMode=Use specified scaling  ParameterScaling=1  OutScaling=1  RndMeth=Nearest  SaturateOnIntegerOverflow=on
  b(4) : Gain  Gain=-0.010230117696056244  ParameterDataTypeMode=Specify via dialog  ParameterDataType=float('double')  ParameterScalingMode=Use specified scaling  ParameterScaling=1  OutScaling=1  RndMeth=Nearest  SaturateOnIntegerOverflow=on
  b(5) : Gain  Gain=-0.024022228586093927  ParameterDataTypeMode=Specify via dialog  ParameterDataType=float('double')  ParameterScalingMode=Use specified scaling  ParameterScaling=1  OutScaling=1  RndMeth=Nearest  SaturateOnIntegerOverflow=on
  b(6) : Gain  Gain=-0.017112476184483319  ParameterDataTypeMode=Specify via dialog  ParameterDataType=float('double')  ParameterScalingMode=Use specified scaling  ParameterScaling=1  OutScaling=1  RndMeth=Nearest  SaturateOnIntegerOverflow=on
  b(7) : Gain  Gain=0.013219031256279611  ParameterDataTypeMode=Specify via dialog  ParameterDataType=float('double')  ParameterScalingMode=Use specified scaling  ParameterScaling=1  OutScaling=1  RndMeth=Nearest  SaturateOnIntegerOverflow=on
  b(8) : Gain  Gain=0.034704857949413304  ParameterDataTypeMode=Specify via dialog  ParameterDataType=float('double')  ParameterScalingMode=Use specified scaling  ParameterScaling=1  OutScaling=1  RndMeth=Nearest  SaturateOnIntegerOverflow=on
  b(9) : Gain  Gain=0.0090330088298889565  ParameterDataTypeMode=Specify via dialog  ParameterDataType=float('double')  ParameterScalingMode=Use specified scaling  ParameterScaling=1  OutScaling=1  RndMeth=Nearest  SaturateOnIntegerOverflow=on
  Output : Outport
  wires:
  Input/1 -> b(1)/1, BodyDelay2/1
  b(1)/1 -> BodyLSum2/2
  BodyDelay2/1 -> b(2)/1, BodyDelay3/1
  b(2)/1 -> BodyLSum2/1
  BodyLSum2/1 -> BodyLSum3/2
  BodyDelay3/1 -> b(3)/1, BodyDelay4/1
  b(3)/1 -> BodyLSum3/1
  BodyLSum3/1 -> BodyLSum4/2
  BodyDelay4/1 -> b(4)/1, BodyDelay5/1
  b(4)/1 -> BodyLSum4/1
  BodyLSum4/1 -> BodyLSum5/2
  BodyDelay5/1 -> b(5)/1, BodyDelay6/1
  b(5)/1 -> BodyLSum5/1
  BodyLSum5/1 -> BodyLSum6/2
  BodyDelay6/1 -> b(6)/1, BodyDelay7/1
  b(6)/1 -> BodyLSum6/1
  BodyLSum6/1 -> BodyLSum7/2
  BodyDelay7/1 -> b(7)/1, BodyDelay8/1
  b(7)/1 -> BodyLSum7/1
  BodyLSum7/1 -> BodyLSum8/2
  BodyDelay8/1 -> b(8)/1, BodyDelay9/1
  b(8)/1 -> BodyLSum8/1
  BodyLSum8/1 -> BodyLSum9/2
  BodyDelay9/1 -> b(9)/1, BodyDelay10/1
  b(9)/1 -> BodyLSum9/1
  BodyLSum9/1 -> BodyLSum10/2
  BodyDelay10/1 -> b(10)/1, BodyDelay11/1
  b(10)/1 -> BodyLSum10/1
  BodyLSum10/1 -> BodyLSum11/2
  BodyDelay11/1 -> b(11)/1, BodyDelay12/1
  b(11)/1 -> BodyLSum11/1
  BodyLSum11/1 -> BodyLSum12/2
  BodyDelay12/1 -> b(12)/1, BodyDelay13/1
  b(12)/1 -> BodyLSum12/1
  BodyLSum12/1 -> BodyLSum13/2
  BodyDelay13/1 -> b(13)/1, BodyDelay14/1
  b(13)/1 -> BodyLSum13/1
  BodyLSum13/1 -> BodyLSum14/2
  BodyDelay14/1 -> b(14)/1, BodyDelay15/1
  b(14)/1 -> BodyLSum14/1
  BodyLSum14/1 -> BodyLSum15/2
  BodyDelay15/1 -> b(15)/1, BodyDelay16/1
  b(15)/1 -> BodyLSum15/1
  BodyLSum15/1 -> BodyLSum16/2
  BodyDelay16/1 -> b(16)/1, BodyDelay17/1
  b(16)/1 -> BodyLSum16/1
  BodyLSum16/1 -> BodyLSum17/2
  BodyDelay17/1 -> b(17)/1, BodyDelay18/1
  b(17)/1 -> BodyLSum17/1
  BodyLSum17/1 -> BodyLSum18/2
  BodyDelay18/1 -> b(18)/1, BodyDelay19/1
  b(18)/1 -> BodyLSum18/1
  BodyLSum18/1 -> BodyLSum19/2
  BodyDelay19/1 -> b(19)/1, BodyDelay20/1
  b(19)/1 -> BodyLSum19/1
  BodyLSum19/1 -> BodyLSum20/2
  BodyDelay20/1 -> b(20)/1, BodyDelay21/1
  b(20)/1 -> BodyLSum20/1
  BodyLSum20/1 -> BodyLSum21/2
  BodyDelay21/1 -> b(21)/1, BodyDelay22/1
  b(21)/1 -> BodyLSum21/1
  BodyLSum21/1 -> BodyLSum22/2
  BodyDelay22/1 -> b(22)/1, BodyDelay23/1
  b(22)/1 -> BodyLSum22/1
  BodyLSum22/1 -> BodyLSum23/2
  BodyDelay23/1 -> b(23)/1, BodyDelay24/1
  b(23)/1 -> BodyLSum23/1
  BodyLSum23/1 -> BodyLSum24/2
  BodyDelay24/1 -> b(24)/1, BodyDelay25/1
  b(24)/1 -> BodyLSum24/1
  BodyLSum24/1 -> BodyLSum25/2
  BodyDelay25/1 -> b(25)/1, BodyDelay26/1
  b(25)/1 -> BodyLSum25/1
  BodyLSum25/1 -> BodyLSum26/2
  BodyDelay26/1 -> b(26)/1, BodyDelay27/1
  b(26)/1 -> BodyLSum26/1
  BodyLSum26/1 -> BodyLSum27/2
  BodyDelay27/1 -> b(27)/1, BodyDelay28/1
  b(27)/1 -> BodyLSum27/1
  BodyLSum27/1 -> BodyLSum28/1
  BodyDelay28/1 -> b(28)/1
  b(28)/1 -> BodyLSum28/2
  BodyLSum28/1 -> Output/1
